simulink model "myexp6"  (R2022a)
settings: Solver=VariableStepAuto  StartTime=0.0  StopTime=100000  RelTol=1e-3
libraries: dspstat3 x2, commchan3 x1, commrandsrc3 x1, commsink2 x1
settings Model: Creator=惠普  LastModifiedBy=惠普

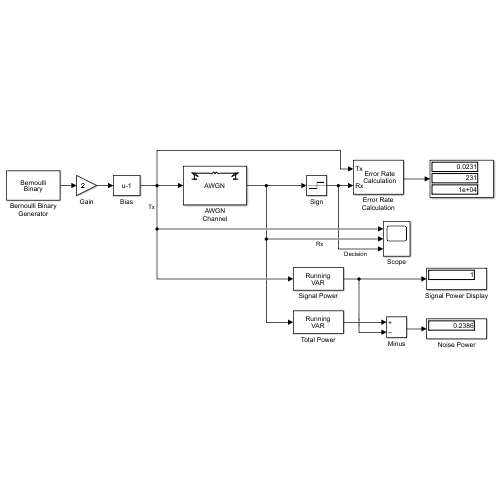
[thumbnail: Simulink's stored preview of the top-level diagram]
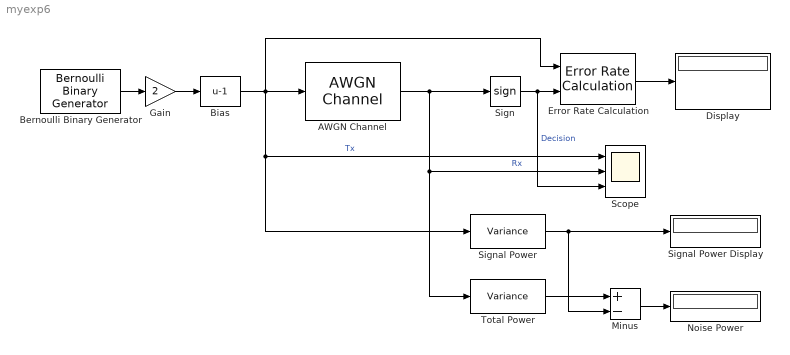
== system myexp6 ==
  AWGN Channel : commchan3/AWGN Channel  InputProcessing=Columns as channels (frame based)  seed=137  noiseMode=Variance from mask  EbNodB=10  EsNodB=10  SNRdB=10  bitsPerSym=1  Ps=1  Tsym=1  variance=0.25
  Bernoulli Binary Generator : commrandsrc3/Bernoulli Binary Generator  ProbabilityOfZero=0.5  SeedSource=Auto  Seed=0  SampleTime=1  SamplesPerFrame=1  OutputDataType=double  SimulateUsing=Interpreted execution
  Bias : Bias  Bias=-1  SaturateOnIntegerOverflow=off
  Display : Display
  Error Rate Calculation : commsink2/Error Rate Calculation  N=0  st_delay=0  cp_mode=Entire frame  subframe=[]  PMode=Port  WsName=ErrorVec  RsMode2=off  stop=off  numErr=100  maxBits=1e6
  Gain : Gain  Gain=2
  Minus : Sum  Inputs=+-
  Noise Power : Display
  Scope : Scope  NumInputPorts=3
  Sign : Signum
  Signal Power : dspstat3/Variance  run=on  InputProcessing=Columns as channels (frame based)  reset_popup=None  directionMode=Each column  dimension=1  roiEnable=off  roiType=Rectangles  roiPortion=Entire ROI  roiOutput=Individual statistics for each ROI  roiFlag=off  roundingMode=Floor  overflowMode=off
  Signal Power Display : Display
  Total Power : dspstat3/Variance  run=on  InputProcessing=Columns as channels (frame based)  reset_popup=None  directionMode=Each column  dimension=1  roiEnable=off  roiType=Rectangles  roiPortion=Entire ROI  roiOutput=Individual statistics for each ROI  roiFlag=off  roundingMode=Floor  overflowMode=off
  wires:
  Bernoulli Binary Generator/1 -> Gain/1
  Gain/1 -> Bias/1
  Bias/1 -> Error Rate Calculation/1, Signal Power/1, Scope/1, AWGN Channel/1  "Tx"
  AWGN Channel/1 -> Total Power/1, Scope/2, Sign/1  "Rx"
  Sign/1 -> Scope/3, Error Rate Calculation/2  "Decision"
  Signal Power/1 -> Minus/2, Signal Power Display/1
  Error Rate Calculation/1 -> Display/1
  Minus/1 -> Noise Power/1
  Total Power/1 -> Minus/1
